simulink model "Simulation_Model_3"  (Simulink 10.1)
settings: Solver=VariableStepAuto  StartTime=0.0  StopTime=70  RelTol=1e-3
settings Model: Creator=Dravius  LastModifiedBy=Roma
settings DataIOCC: SaveFormat=Dataset
settings OptimizationCC: LifeSpan=auto
settings DebuggingCC: UnderspecifiedInitializationDetection=Simplified  MergeDetectMultiDrivingBlocksExec=error  SFUnexpectedBacktrackingDiag=error  SFNoUnconditionalDefaultTransitionDiag=error  SFExecutionAtInitializationDiag=warning
settings HardwareCC: ProdBitPerPointer=64  ProdBitPerSizeT=64  ProdBitPerPtrDiffT=64  ProdLargestAtomicFloat=Float  ProdIntDivRoundTo=Zero  ProdEndianess=LittleEndian  ProdWordSize=64  ProdHWDeviceType=Intel->x86-64 (Windows64)
settings ModelReferenceCC: PropagateSignalLabelsOutOfModel=on
settings SFSimCC: SimUseLocalCustomCode=on
settings RTWCC: RTWUseLocalCustomCode=on
settings CodeAppCC: StateflowObjectComments=off
settings GRTTargetCC: TargetLangStandard=C99 (ISO)  CombineOutputUpdateFcns=on  GRTInterface=off
settings ConfigComp: CovMetricSettings=dwe  CovHtmlReporting=off  CovSaveCumulativeToWorkspaceVar=off  CovSaveSingleToWorkspaceVar=off  CovExternalEMLEnable=on

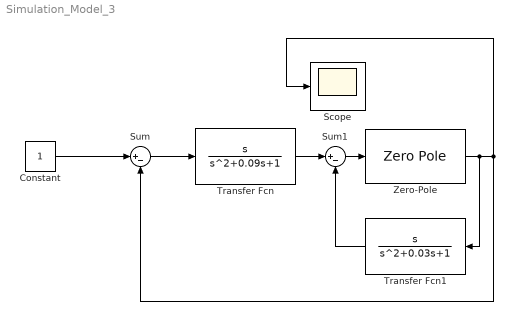
== system Simulation_Model_3 ==
  Constant : Constant
  Scope : Scope
  Sum : Sum  Inputs=|+-
  Sum1 : Sum  Inputs=|+-
  Transfer Fcn : TransferFcn  Numerator=[1 0]  Denominator=[1 0.09 1]
  Transfer Fcn1 : TransferFcn  Numerator=[1 0]  Denominator=[1 0.03 1]
  Zero-Pole : ZeroPole  Zeros=[0]  Poles=[-0.06 -1]
  wires:
  Constant/1 -> Sum/1
  Sum/1 -> Transfer Fcn/1
  Transfer Fcn/1 -> Sum1/1
  Sum1/1 -> Zero-Pole/1
  Zero-Pole/1 -> Transfer Fcn1/1, Sum/2, Scope/1
  Transfer Fcn1/1 -> Sum1/2
